simulink model "AdaptiveandRRTxBackstepping21a"  (R2022a)
settings: Solver=ode1  StartTime=0.0  StopTime=30  FixedStep=0.01  RelTol=1e-3  EnableMultiTasking=on
undefined symbols (not defined in the file): ux, uy
libraries: arduinolib x5, arduinosensorlib x1, mobileRoboticsLib x1
(part 2 of 2)

== matlab function AdaptiveandRRTxBackstepping21a/MATLAB Function16 ==
  settings: updateMethod=DISCRETE
  data: uk input; y_true input; x_est output
function x_est = ekf(uk,y_true)
Ts = 0.01;
persistent x_est_p P Qd_est R_est Qc_est;
if isempty(x_est_p)
    x_est_p = [0;0;0;0];
    P       = 1e-0*diag([10,1,30,1]);
    Qc_est  = 1e-4*diag([1,10,100,10]);
    Qd_est  = Ts*Qc_est;
    R_est   = 0.001;
end
c  = [1 0 0 0];
D  = 0;
Ck = c;
Dk = D;

%Comput Kalman Gain and update predicted value
Wk    = P*Ck'/(Ck*P*Ck'+R_est);
y_est = Ck*x_est_p+Dk*uk;
x     = x_est_p+Wk.*(y_true-y_est);

%Compute prediction at next time step
x_est = x+Ts*[-x(2)*x(1)+uk*x(3)-x(4)*sign(x(1));
                          0;
                          0;
                          0];

%Update error covariance matrices
P = P-Wk*Ck*P;

%Define Ak
Ak      = eye(4)+Ts*[-x(2) -x(1) uk -sign(x(1));
                 0     0    0      0;
                 0     0    0      0;
                 0     0    0      0];
P       = Ak*P*Ak'+Qd_est;
x_est_p = x_est;

== matlab function AdaptiveandRRTxBackstepping21a/MATLAB Function17 ==
  data: a output; b output; c output; t input; a_nw input; b_nw input; c_nw input
function [a,b,c] = fcn(t,a_nw,b_nw,c_nw)

a = 28.37;
b = 19.15;
c = 5.75;

if t>0.5
a = a_nw;
b = b_nw;
c = c_nw;
end

== matlab function AdaptiveandRRTxBackstepping21a/MATLAB Function1 ==
  data: Xd_dot input; v_d output; w_d output
function [v_d, w_d] = fcn(Xd_dot)
% convert velocity in global frame to body frame. No need rotation matrix just need projection.
v_d = sqrt(Xd_dot(1)^2 + Xd_dot(2)^2);
w_d = Xd_dot(3);

== matlab function AdaptiveandRRTxBackstepping21a/MATLAB Function2 ==
  settings: updateMethod=DISCRETE
  data: t input; route input; x_d input; y_d input; theta_d input; X_r_dot output; X input; V_max output; omega_max output; X_W_c input
function [X_r_dot, V_max, omega_max]   = fcn(t,route,x_d,y_d,theta_d, X, X_W_c)
%#codegen

persistent k i j X_p_i omega_p_j t1 t2
if isempty(k)
    i = int8(1);
    j = int8(1);
    X_p_i = [0;0];
    omega_p_j = 0;
    t1 = t;
    t2 = t;
    k = 1;
end
tau = 0.15;
tau1 = 0.15;
V_max = 0.3; % maximum velocity0.6
a = 3;      % acceleration5
omega_max = 2; %2
alpha = 1; %1

X_r_dot = zeros(3,1);
switch route
    case 1
%         X_p = [1.5   1.5  0];
%%%%%%%%%%%%%theta_d = zeros(length(x),1);
        X_p = [x_d,y_d,theta_d]; % X_p = [x,y,theta];
    otherwise
        X_r_dot = [0;0;0];
        return;
end
X_p = X_p'; % X_p = [x;y;theta]
[~,col] = size(X_p);
dX = X_p(1:2,i)-X_p_i;
norm_dX = norm(dX);
two_rmin = V_max^2/a;  
dtheta = X_p(3,j)-omega_p_j;
norm_dtheta = abs(dtheta);
two_thetamin = omega_max^2/alpha; 

if norm_dX > two_rmin
    ta = V_max/a;                   % acceleration period
    tad = (norm_dX-two_rmin)/V_max; % acc to deceleration period
    td = ta + tad;                  % start deceleration
    te = ta + td;                   % end deceleration
    if (t-t1) < ta
        v = a*(t-t1);
    elseif ta <= (t-t1) && (t-t1) < td
        v = V_max;
    elseif td <= (t-t1) && (t-t1) < te
        v = -a*(t-t1-td) + V_max;
    else
        v = 0;
    end
else
    tp = sqrt(norm_dX/a);
    te = 2*tp;
    Vp = a*tp;
    if (t-t1) < tp
        v = a*(t-t1);
    elseif tp < (t-t1) && (t-t1) < te
        v = -a*(t-t1-tp)+Vp;
    else
        v = 0;
    end
end
if norm_dX~=0
    X_r_dot(1:2) = v*dX/norm_dX;
end

dist_X = norm(X_p(1:2,i)-X(1:2));
if (i<col)&&(dist_X < tau)
    X_p_i = X(1:2);
    t1    = t;
    i     = i+1;
end

if norm_dtheta > two_thetamin
    ta = omega_max/alpha;                   % acceleration period
    tad = (norm_dtheta-two_thetamin)/omega_max; % acc to deceleration period
    td = ta + tad;                  % start deceleration
    te = ta + td;                   % end deceleration
    if (t-t2) < ta
        omega = alpha*(t-t2);
    elseif ta <= (t-t2) && (t-t2) < td
        omega = omega_max;
    elseif td <= (t-t2) && (t-t2) < te
        omega = -alpha*(t-t2-td) + omega_max;
    else
        omega = 0;
    end
else
    tp = sqrt(norm_dtheta/alpha);
    te = 2*tp;
    omegap = alpha*tp;
    if (t-t2) < tp
        omega = alpha*(t-t2);
    elseif tp < (t-t2) && (t-t2) < te
        omega = -alpha*(t-t2-tp)+omegap;
    else
        % only control the orientation at final point, oemga = 2*(X_W_c(3) - X_p(3,end))
        % if not final point, no need to control the orientation, so omega = 0
        e_x = abs(X_W_c(1) - X_p(1,end));
        e_y = abs(X_W_c(2) - X_p(2,end));
        e_theta = X_W_c(3) - X_p(3,end);
        if  e_x < 0.5 && e_y < 0.5 && abs(e_theta) > 1*pi/180
        omega = 0.8*(X_W_c(3) - X_p(3,end));
        else
        omega = 0;
        end
    end
end
X_r_dot(3) = omega*sign(dtheta);

%Generate w to control final point orientation
%e_x = abs(X_W_c(1) - X_p(1,end));
%e_y = abs(X_W_c(2) - X_p(2,end));
%e_theta = X_W_c(3) - X_p(3,end);
%if  e_x < 0.5 && e_y < 0.5 && abs(e_theta) > 3*pi/180
 %   omega = -2*(X_W_c(3) - X_p(3,end));
%elseif e_x < 0.5 && e_y < 0.5 && abs(e_theta) <= 3*pi/180
 %   omega = 0;
%end
%X_r_dot(3) = omega;

dist_theta = abs(X_p(3,j)-X(3));
if (j<col)&&(dist_theta < tau1)
    omega_p_j = X(3);
    t2    = t;
    j     = j+1;
end
